simulink model "lead_steady_then_slow"  (R2025a)
settings: Solver=VariableStepAuto  StartTime=0.0  StopTime=20.0  RelTol=1e-3
settings Model: Creator=sanborkl  LastModifiedBy=sanborkl

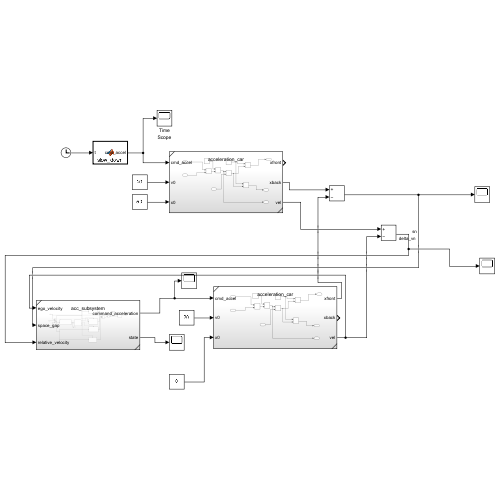
[thumbnail: Simulink's stored preview of the top-level diagram]
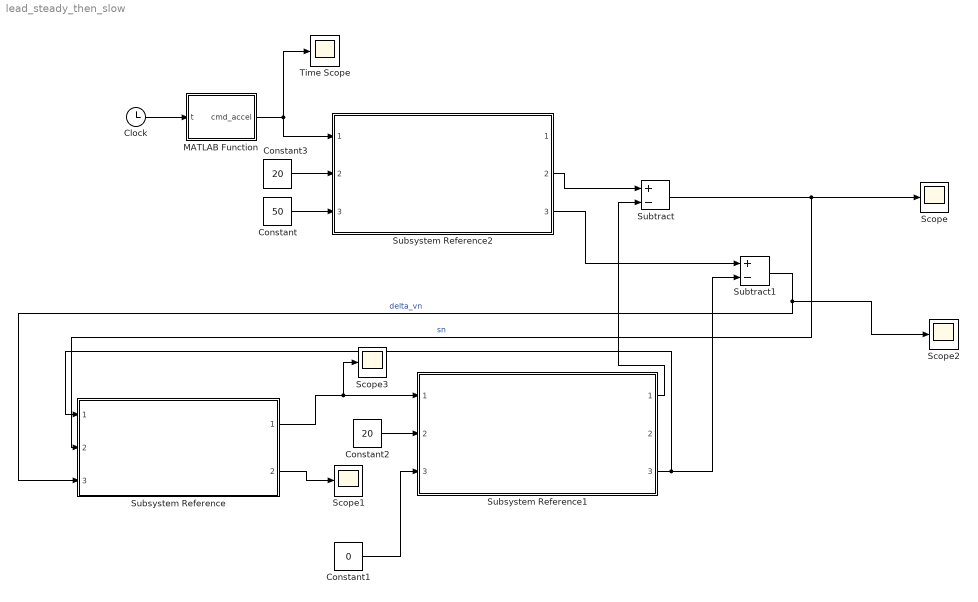
== system lead_steady_then_slow ==
  Clock : Clock
  Constant : Constant  Value=50
  Constant1 : Constant  Value=0
  Constant2 : Constant  Value=20
  Constant3 : Constant  Value=20
  MATLAB Function : MATLAB Function  TreatAsAtomicUnit=on
  Scope{,1..3} (4 alike) : Scope
      Scope settings: ActiveDisplayYMinimum=7.0577298305674168  ActiveDisplayYMaximum=50.060252241048069
      Scope1 settings: ActiveDisplayYMinimum=-1  ActiveDisplayYMaximum=1  DataLoggingVariableName=ScopeData2
      Scope2 settings: ActiveDisplayYMinimum=-1  ActiveDisplayYMaximum=1  DataLoggingVariableName=ScopeData3
      Scope3 settings: ActiveDisplayYMinimum=-1.6601447210305178  ActiveDisplayYMaximum=1.8511271912256131  DataLoggingVariableName=ScopeData4
  Subsystem Reference : Subsystem  ReferencedSubsystem=acc_subsystem
  Subsystem Reference1 : Subsystem  ReferencedSubsystem=acceleration_car
  Subsystem Reference2 : Subsystem  ReferencedSubsystem=acceleration_car
  Subtract : Sum  Inputs=+-
  Subtract1 : Sum  Inputs=+-
  Time Scope : Scope
      settings: TimeUnits=Metric (based on Time Span)  ActiveDisplayYMinimum=-1.125  ActiveDisplayYMaximum=0.12499999999999997  YLabel=Amplitude
  wires:
  Subsystem Reference/1 -> Scope3/1, Subsystem Reference1/1
  Subsystem Reference2/2 -> Subtract/1
  Subsystem Reference1/1 -> Subtract/2
  Subtract/1 -> Subsystem Reference/2, Scope/1  "sn"
  Subsystem Reference2/3 -> Subtract1/1
  Subsystem Reference1/3 -> Subsystem Reference/1, Subtract1/2
  Subtract1/1 -> Scope2/1, Subsystem Reference/3  "delta_vn"
  Constant/1 -> Subsystem Reference2/3
  Constant1/1 -> Subsystem Reference1/3
  Constant2/1 -> Subsystem Reference1/2
  Clock/1 -> MATLAB Function/1(t)
  MATLAB Function/1(cmd_accel) -> Subsystem Reference2/1, Time Scope/1
  Subsystem Reference/2 -> Scope1/1
  Constant3/1 -> Subsystem Reference2/2

== matlab function lead_steady_then_slow/MATLAB Function ==
  data: t input; cmd_accel output
function cmd_accel = slow_down(t)

if t < 4
    cmd_accel = 0;
else
    cmd_accel = -1;
end
